simulink model "filtro_media_movel_2"  (R2019b)
settings: Solver=VariableStepAuto  StartTime=0.0  StopTime=10.0  RelTol=1e-3
values from neighbouring files (symbols this model uses):
  T = 0.00833333333333    [ECG_graficos_fft.mat]    (also in FPB_Arduino.mat = 0.001; butter1.mat = 1.25e-08; filtro_notch1.mat; intro_resp_freq.mat = 0.00125)
settings Model: Creator=fernandopassold  LastModifiedBy=fernandopassold

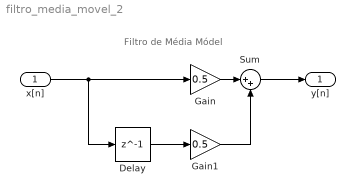
== system filtro_media_movel_2 ==
  note: Filtro de Média Módel
  x[n] : Inport
  Delay : Delay  DelayLength=1  SampleTime=T
  Gain : Gain  Gain=0.5
  Gain1 : Gain  Gain=0.5
  Sum : Sum  Inputs=|++
  y[n] : Outport
  wires:
  x[n]/1 -> Delay/1, Gain/1
  Gain/1 -> Sum/1
  Sum/1 -> y[n]/1
  Delay/1 -> Gain1/1
  Gain1/1 -> Sum/2
